simulink model "Charge_2_V1"  (R2017b)
settings: Solver=FixedStepDiscrete  StartTime=0.0  StopTime=1  FixedStep=0.001  RelTol=1e-3
PreLoadFcn:
  | librarySetup
  | eval([bdroot,'_startup']) %Calling [modelName]_startup.m
undefined symbols (not defined in the file or in its folder): A0, A1, Car1__Authorize, Car2_Authorize, CON2, CON3, CON4, Control_Mode_In, CurrentSP, D10, D12, D13, D2, D3, D4, D5, D6, D7, D8, Frequency_High_Point, Frequency_Low_Point, Frequency_Mid_high, Frequency_Mid_low, HVol_High_Point, HVol_Low_Point, HVol_Mid_high, HVol_Mid_low, HVoltage_Factor, SeconCar_ThreePhase, V_Current_five, V_Current_four, V_Current_one, V_Current_six, V_Current_three, V_Current_two, V_Frequency, V_MaxPliot, V_MinPliot, Vol_High_Point, Vol_Low_Point, Vol_Mid_high, Vol_Mid_low, Voltage_Factor, Voltage_Mode_Test
libraries: simulink x331, HANcoder_STM32_Target x30, powerlib_meascontrol x8, simulink_extras x2
(part 3 of 13)

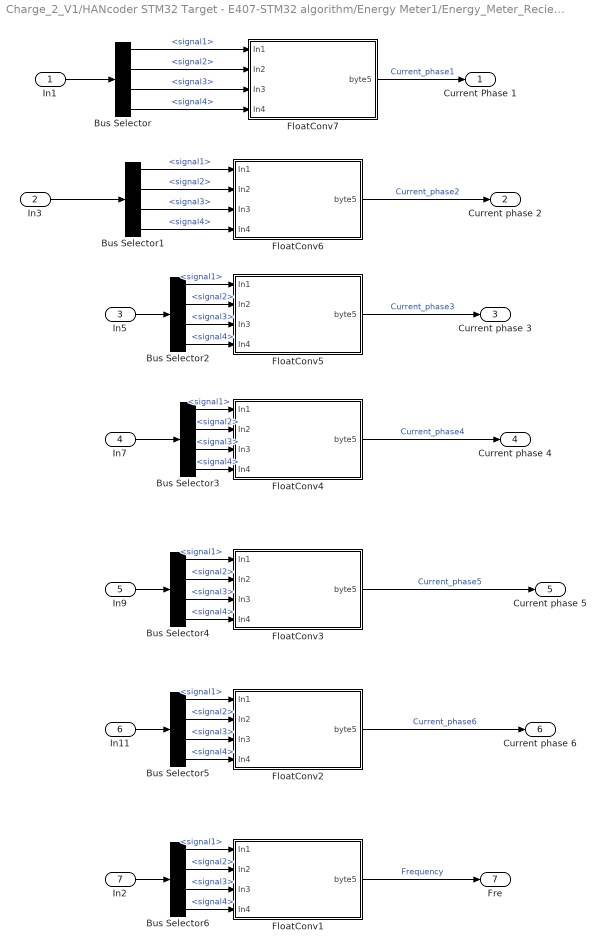
== system Charge_2_V1/HANcoder STM32 Target - E407-STM32 algorithm/Energy Meter1/Energy_Meter_Recieve/Subsystem ==
  In1 : Inport  SampleTime=0.1
  In3 : Inport  Port=2  SampleTime=0.1
  In5 : Inport  Port=3  SampleTime=0.1
  In7 : Inport  Port=4  SampleTime=0.1
  In9 : Inport  Port=5  SampleTime=0.1
  In11 : Inport  Port=6  SampleTime=0.1
  In2 : Inport  Port=7  SampleTime=0.1
  Bus Selector{,1..6} (7 alike) : BusSelector  OutputSignals=signal1,signal2,signal3,signal4
  FloatConv1 : Subsystem
  FloatConv2 : Subsystem
  FloatConv3 : Subsystem
  FloatConv4 : Subsystem
  FloatConv5 : Subsystem
  FloatConv6 : Subsystem
  FloatConv7 : Subsystem
  Current Phase 1 : Outport
  Current phase 2 : Outport  Port=2  SampleTime=0.1
  Current phase 3 : Outport  Port=3  SampleTime=0.1
  Current phase 4 : Outport  Port=4  SampleTime=0.1
  Current phase 5 : Outport  Port=5  SampleTime=0.1
  Current phase 6 : Outport  Port=6  SampleTime=0.1
  Fre : Outport  Port=7  SampleTime=0.1
  wires:
  FloatConv7/1(byte5) -> Current Phase 1/1  "Current_phase1"
  FloatConv6/1(byte5) -> Current phase 2/1  "Current_phase2"
  FloatConv5/1(byte5) -> Current phase 3/1  "Current_phase3"
  FloatConv4/1(byte5) -> Current phase 4/1  "Current_phase4"
  FloatConv3/1(byte5) -> Current phase 5/1  "Current_phase5"
  FloatConv2/1(byte5) -> Current phase 6/1  "Current_phase6"
  FloatConv1/1(byte5) -> Fre/1  "Frequency"
  In1/1 -> Bus Selector/1
  Bus Selector/1 -> FloatConv7/1(In1)  "<signal1>"
  Bus Selector/2 -> FloatConv7/2(In2)  "<signal2>"
  Bus Selector/3 -> FloatConv7/3(In3)  "<signal3>"
  Bus Selector/4 -> FloatConv7/4(In4)  "<signal4>"
  In3/1 -> Bus Selector1/1
  Bus Selector1/1 -> FloatConv6/1(In1)  "<signal1>"
  Bus Selector1/2 -> FloatConv6/2(In2)  "<signal2>"
  Bus Selector1/3 -> FloatConv6/3(In3)  "<signal3>"
  Bus Selector1/4 -> FloatConv6/4(In4)  "<signal4>"
  Bus Selector2/1 -> FloatConv5/1(In1)  "<signal1>"
  Bus Selector2/2 -> FloatConv5/2(In2)  "<signal2>"
  Bus Selector2/3 -> FloatConv5/3(In3)  "<signal3>"
  Bus Selector2/4 -> FloatConv5/4(In4)  "<signal4>"
  In5/1 -> Bus Selector2/1
  Bus Selector3/1 -> FloatConv4/1(In1)  "<signal1>"
  Bus Selector3/2 -> FloatConv4/2(In2)  "<signal2>"
  Bus Selector3/3 -> FloatConv4/3(In3)  "<signal3>"
  Bus Selector3/4 -> FloatConv4/4(In4)  "<signal4>"
  In7/1 -> Bus Selector3/1
  In9/1 -> Bus Selector4/1
  Bus Selector4/1 -> FloatConv3/1(In1)  "<signal1>"
  Bus Selector4/2 -> FloatConv3/2(In2)  "<signal2>"
  Bus Selector4/3 -> FloatConv3/3(In3)  "<signal3>"
  Bus Selector4/4 -> FloatConv3/4(In4)  "<signal4>"
  Bus Selector5/1 -> FloatConv2/1(In1)  "<signal1>"
  Bus Selector5/2 -> FloatConv2/2(In2)  "<signal2>"
  Bus Selector5/3 -> FloatConv2/3(In3)  "<signal3>"
  Bus Selector5/4 -> FloatConv2/4(In4)  "<signal4>"
  In11/1 -> Bus Selector5/1
  In2/1 -> Bus Selector6/1
  Bus Selector6/1 -> FloatConv1/1(In1)  "<signal1>"
  Bus Selector6/2 -> FloatConv1/2(In2)  "<signal2>"
  Bus Selector6/3 -> FloatConv1/3(In3)  "<signal3>"
  Bus Selector6/4 -> FloatConv1/4(In4)  "<signal4>"

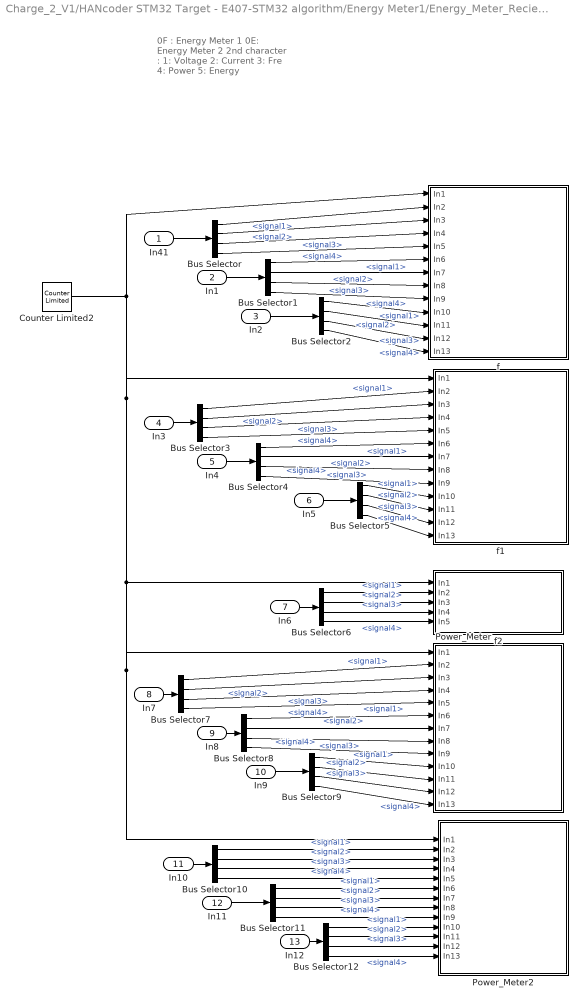
== system Charge_2_V1/HANcoder STM32 Target - E407-STM32 algorithm/Energy Meter1/Energy_Meter_Recieve/Subsystem1 ==
  note: 0F : Energy Meter 1
      | 0E: Energy Meter 2
      | 2nd character :
      | 1: Voltage
      | 2: Current
      | 3: Fre
      | 4: Power
      | 5: Energy
  In41 : Inport
  In1 : Inport  Port=2
  In2 : Inport  Port=3
  In3 : Inport  Port=4
  In4 : Inport  Port=5
  In5 : Inport  Port=6
  In6 : Inport  Port=7
  In7 : Inport  Port=8
  In8 : Inport  Port=9
  In9 : Inport  Port=10
  In10 : Inport  Port=11
  In11 : Inport  Port=12
  In12 : Inport  Port=13
  Bus Selector{,1..12} (13 alike) : BusSelector  OutputSignals=signal1,signal2,signal3,signal4
  Counter Limited2 : simulink/Sources/Counter Limited  uplimit=1200  tsamp=0.001
  Power_Meter : Subsystem
  Power_Meter2 : Subsystem
  f : Subsystem
  f1 : Subsystem
  f2 : Subsystem
  wires:
  Counter Limited2/1 -> f/1(In1), Power_Meter2/1(In1), Power_Meter/1(In1), f2/1(In1), f1/1(In1)
  In41/1 -> Bus Selector/1
  Bus Selector/1 -> f/2(In2)  "<signal1>"
  Bus Selector/2 -> f/3(In3)  "<signal2>"
  Bus Selector/3 -> f/4(In4)  "<signal3>"
  Bus Selector/4 -> f/5(In5)  "<signal4>"
  In1/1 -> Bus Selector1/1
  Bus Selector1/1 -> f/6(In6)  "<signal1>"
  Bus Selector1/2 -> f/7(In7)  "<signal2>"
  Bus Selector1/3 -> f/8(In8)  "<signal3>"
  Bus Selector1/4 -> f/9(In9)  "<signal4>"
  Bus Selector2/1 -> f/10(In10)  "<signal1>"
  Bus Selector2/2 -> f/11(In11)  "<signal2>"
  Bus Selector2/3 -> f/12(In12)  "<signal3>"
  Bus Selector2/4 -> f/13(In13)  "<signal4>"
  In2/1 -> Bus Selector2/1
  Bus Selector3/1 -> f1/2(In2)  "<signal1>"
  Bus Selector3/2 -> f1/3(In3)  "<signal2>"
  Bus Selector3/3 -> f1/4(In4)  "<signal3>"
  Bus Selector3/4 -> f1/5(In5)  "<signal4>"
  In3/1 -> Bus Selector3/1
  Bus Selector4/1 -> f1/6(In6)  "<signal1>"
  Bus Selector4/2 -> f1/7(In7)  "<signal2>"
  Bus Selector4/3 -> f1/8(In8)  "<signal3>"
  Bus Selector4/4 -> f1/9(In9)  "<signal4>"
  In4/1 -> Bus Selector4/1
  Bus Selector5/2 -> f1/11(In11)  "<signal2>"
  Bus Selector5/3 -> f1/12(In12)  "<signal3>"
  Bus Selector5/4 -> f1/13(In13)  "<signal4>"
  Bus Selector5/1 -> f1/10(In10)  "<signal1>"
  In5/1 -> Bus Selector5/1
  In6/1 -> Bus Selector6/1
  Bus Selector7/1 -> Power_Meter/2(In2)  "<signal1>"
  Bus Selector7/2 -> Power_Meter/3(In3)  "<signal2>"
  Bus Selector7/3 -> Power_Meter/4(In4)  "<signal3>"
  Bus Selector7/4 -> Power_Meter/5(In5)  "<signal4>"
  Bus Selector8/1 -> Power_Meter/6(In6)  "<signal1>"
  Bus Selector8/2 -> Power_Meter/7(In7)  "<signal2>"
  Bus Selector8/3 -> Power_Meter/8(In8)  "<signal3>"
  Bus Selector8/4 -> Power_Meter/9(In9)  "<signal4>"
  Bus Selector9/1 -> Power_Meter/10(In10)  "<signal1>"
  Bus Selector9/2 -> Power_Meter/11(In11)  "<signal2>"
  Bus Selector9/3 -> Power_Meter/12(In12)  "<signal3>"
  Bus Selector9/4 -> Power_Meter/13(In13)  "<signal4>"
  In7/1 -> Bus Selector7/1
  In8/1 -> Bus Selector8/1
  In9/1 -> Bus Selector9/1
  Bus Selector11/1 -> Power_Meter2/6(In6)  "<signal1>"
  Bus Selector11/2 -> Power_Meter2/7(In7)  "<signal2>"
  Bus Selector11/3 -> Power_Meter2/8(In8)  "<signal3>"
  Bus Selector11/4 -> Power_Meter2/9(In9)  "<signal4>"
  Bus Selector12/1 -> Power_Meter2/10(In10)  "<signal1>"
  Bus Selector12/2 -> Power_Meter2/11(In11)  "<signal2>"
  Bus Selector12/3 -> Power_Meter2/12(In12)  "<signal3>"
  Bus Selector12/4 -> Power_Meter2/13(In13)  "<signal4>"
  In10/1 -> Bus Selector10/1
  In11/1 -> Bus Selector11/1
  In12/1 -> Bus Selector12/1
  Bus Selector6/1 -> f2/2(In2)  "<signal1>"
  Bus Selector6/2 -> f2/3(In3)  "<signal2>"
  Bus Selector6/3 -> f2/4(In4)  "<signal3>"
  Bus Selector6/4 -> f2/5(In5)  "<signal4>"
  Bus Selector10/1 -> Power_Meter2/2(In2)  "<signal1>"
  Bus Selector10/2 -> Power_Meter2/3(In3)  "<signal2>"
  Bus Selector10/3 -> Power_Meter2/4(In4)  "<signal3>"
  Bus Selector10/4 -> Power_Meter2/5(In5)  "<signal4>"

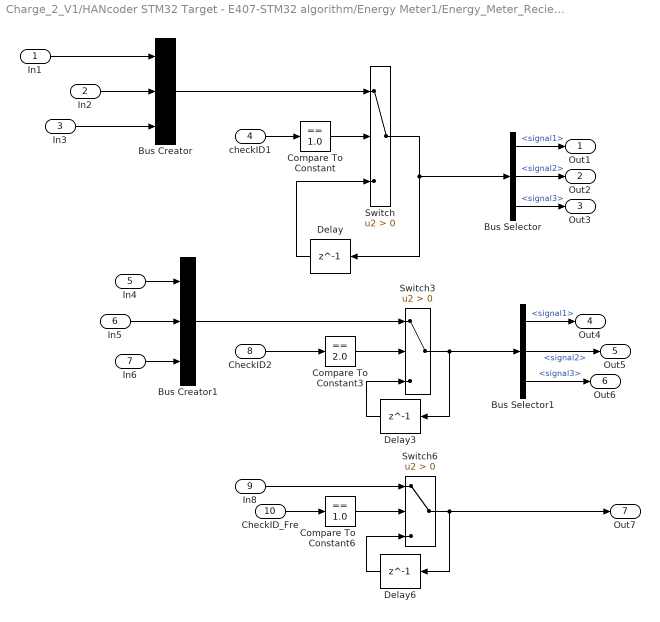
== system Charge_2_V1/HANcoder STM32 Target - E407-STM32 algorithm/Energy Meter1/Energy_Meter_Recieve/Subsystem2 ==
  In1 : Inport
  In2 : Inport  Port=2
  In3 : Inport  Port=3
  checkID1 : Inport  Port=4
  In4 : Inport  Port=5
  In5 : Inport  Port=6
  In6 : Inport  Port=7
  CheckID2 : Inport  Port=8
  In8 : Inport  Port=9
  CheckID_Fre : Inport  Port=10
  Bus Creator : BusCreator  Inputs=3
  Bus Creator1 : BusCreator  Inputs=3
  Bus Selector : BusSelector  OutputSignals=signal1,signal2,signal3
  Bus Selector1 : BusSelector  OutputSignals=signal1,signal2,signal3
  Compare To Constant : simulink/Logic and Bit Operations/Compare To Constant  relop===  const=1.0  OutDataTypeStr=boolean
  Compare To Constant3 : simulink/Logic and Bit Operations/Compare To Constant  relop===  const=2.0  OutDataTypeStr=boolean
  Compare To Constant6 : simulink/Logic and Bit Operations/Compare To Constant  relop===  const=1.0  OutDataTypeStr=boolean
  Delay : Delay  DelayLength=1  InitialCondition=0
  Delay3 : Delay  DelayLength=1  InitialCondition=0
  Delay6 : Delay  DelayLength=1  InitialCondition=0
  Switch : Switch  Criteria=u2 > Threshold
  Switch3 : Switch  Criteria=u2 > Threshold
  Switch6 : Switch  Criteria=u2 > Threshold
  Out1 : Outport
  Out2 : Outport  Port=2
  Out3 : Outport  Port=3
  Out4 : Outport  Port=4
  Out5 : Outport  Port=5
  Out6 : Outport  Port=6
  Out7 : Outport  Port=7
  wires:
  Compare To Constant/1 -> Switch/2
  Switch/1 -> Delay/1, Bus Selector/1
  In1/1 -> Bus Creator/1
  Delay/1 -> Switch/3
  Switch3/1 -> Delay3/1, Bus Selector1/1
  Compare To Constant3/1 -> Switch3/2
  Delay3/1 -> Switch3/3
  Switch6/1 -> Out7/1, Delay6/1
  Compare To Constant6/1 -> Switch6/2
  Delay6/1 -> Switch6/3
  In2/1 -> Bus Creator/2
  In3/1 -> Bus Creator/3
  Bus Creator/1 -> Switch/1
  Bus Creator1/1 -> Switch3/1
  checkID1/1 -> Compare To Constant/1
  In8/1 -> Switch6/1
  Bus Selector/1 -> Out1/1  "<signal1>"
  Bus Selector/2 -> Out2/1  "<signal2>"
  Bus Selector/3 -> Out3/1  "<signal3>"
  In4/1 -> Bus Creator1/1
  In5/1 -> Bus Creator1/2
  In6/1 -> Bus Creator1/3
  CheckID2/1 -> Compare To Constant3/1
  CheckID_Fre/1 -> Compare To Constant6/1
  Bus Selector1/1 -> Out4/1  "<signal1>"
  Bus Selector1/2 -> Out5/1  "<signal2>"
  Bus Selector1/3 -> Out6/1  "<signal3>"

== system Charge_2_V1/HANcoder STM32 Target - E407-STM32 algorithm/Energy Meter1/Energy_Meter_Recieve/Subsystem3 ==
  In1 : Inport
  In2 : Inport  Port=2
  In3 : Inport  Port=3
  checkID1 : Inport  Port=4
  In4 : Inport  Port=5
  In5 : Inport  Port=6
  In6 : Inport  Port=7
  CheckID2 : Inport  Port=8
  Bus Creator : BusCreator  Inputs=3
  Bus Creator1 : BusCreator  Inputs=3
  Bus Selector : BusSelector  OutputSignals=signal1,signal2,signal3
  Bus Selector1 : BusSelector  OutputSignals=signal1,signal2,signal3
  Compare To Constant : simulink/Logic and Bit Operations/Compare To Constant  relop===  const=1.0  OutDataTypeStr=boolean
  Compare To Constant3 : simulink/Logic and Bit Operations/Compare To Constant  relop===  const=2.0  OutDataTypeStr=boolean
  Delay : Delay  DelayLength=1  InitialCondition=0
  Delay3 : Delay  DelayLength=1  InitialCondition=0
  Switch : Switch  Criteria=u2 > Threshold
  Switch3 : Switch  Criteria=u2 > Threshold
  Out1 : Outport
  Out2 : Outport  Port=2
  Out3 : Outport  Port=3
  Out4 : Outport  Port=4
  Out5 : Outport  Port=5
  Out6 : Outport  Port=6
  wires:
  Compare To Constant/1 -> Switch/2
  Switch/1 -> Delay/1, Bus Selector/1
  In1/1 -> Bus Creator/1
  Delay/1 -> Switch/3
  Switch3/1 -> Delay3/1, Bus Selector1/1
  Compare To Constant3/1 -> Switch3/2
  Delay3/1 -> Switch3/3
  In2/1 -> Bus Creator/2
  In3/1 -> Bus Creator/3
  Bus Creator/1 -> Switch/1
  Bus Creator1/1 -> Switch3/1
  checkID1/1 -> Compare To Constant/1
  Bus Selector/1 -> Out1/1  "<signal1>"
  Bus Selector/2 -> Out2/1  "<signal2>"
  Bus Selector/3 -> Out3/1  "<signal3>"
  In4/1 -> Bus Creator1/1
  In5/1 -> Bus Creator1/2
  In6/1 -> Bus Creator1/3
  CheckID2/1 -> Compare To Constant3/1
  Bus Selector1/1 -> Out4/1  "<signal1>"
  Bus Selector1/2 -> Out5/1  "<signal2>"
  Bus Selector1/3 -> Out6/1  "<signal3>"

== system Charge_2_V1/HANcoder STM32 Target - E407-STM32 algorithm/Energy Meter1/Energy_Meter_Recieve/Subsystem5 ==
  In1 : Inport  SampleTime=0.1
  In3 : Inport  Port=2  SampleTime=0.1
  In5 : Inport  Port=3  SampleTime=0.1
  In7 : Inport  Port=4  SampleTime=0.1
  In9 : Inport  Port=5  SampleTime=0.1
  In11 : Inport  Port=6  SampleTime=0.1
  Bus Selector{,1..5} (6 alike) : BusSelector  OutputSignals=signal1,signal2,signal3,signal4
  FloatConv2 : Subsystem
  FloatConv3 : Subsystem
  FloatConv4 : Subsystem
  FloatConv5 : Subsystem
  FloatConv6 : Subsystem
  FloatConv7 : Subsystem
  Voltage1 : Outport
  Voltage2 : Outport  Port=2  SampleTime=0.1
  Voltage3 : Outport  Port=3  SampleTime=0.1
  Voltage4 : Outport  Port=4  SampleTime=0.1
  Voltage5 : Outport  Port=5  SampleTime=0.1
  Voltage6 : Outport  Port=6  SampleTime=0.1
  wires:
  In11/1 -> Bus Selector5/1
  Bus Selector5/4 -> FloatConv2/4(In4)  "<signal4>"
  Bus Selector5/3 -> FloatConv2/3(In3)  "<signal3>"
  Bus Selector5/2 -> FloatConv2/2(In2)  "<signal2>"
  Bus Selector5/1 -> FloatConv2/1(In1)  "<signal1>"
  Bus Selector4/4 -> FloatConv3/4(In4)  "<signal4>"
  Bus Selector4/3 -> FloatConv3/3(In3)  "<signal3>"
  Bus Selector4/2 -> FloatConv3/2(In2)  "<signal2>"
  Bus Selector4/1 -> FloatConv3/1(In1)  "<signal1>"
  In9/1 -> Bus Selector4/1
  In7/1 -> Bus Selector3/1
  Bus Selector3/4 -> FloatConv4/4(In4)  "<signal4>"
  Bus Selector3/3 -> FloatConv4/3(In3)  "<signal3>"
  Bus Selector3/2 -> FloatConv4/2(In2)  "<signal2>"
  Bus Selector3/1 -> FloatConv4/1(In1)  "<signal1>"
  In5/1 -> Bus Selector2/1
  Bus Selector2/4 -> FloatConv5/4(In4)  "<signal4>"
  Bus Selector2/3 -> FloatConv5/3(In3)  "<signal3>"
  Bus Selector2/2 -> FloatConv5/2(In2)  "<signal2>"
  Bus Selector2/1 -> FloatConv5/1(In1)  "<signal1>"
  Bus Selector1/4 -> FloatConv6/4(In4)  "<signal4>"
  Bus Selector1/3 -> FloatConv6/3(In3)  "<signal3>"
  Bus Selector1/2 -> FloatConv6/2(In2)  "<signal2>"
  Bus Selector1/1 -> FloatConv6/1(In1)  "<signal1>"
  In3/1 -> Bus Selector1/1
  Bus Selector/4 -> FloatConv7/4(In4)  "<signal4>"
  Bus Selector/3 -> FloatConv7/3(In3)  "<signal3>"
  Bus Selector/2 -> FloatConv7/2(In2)  "<signal2>"
  Bus Selector/1 -> FloatConv7/1(In1)  "<signal1>"
  In1/1 -> Bus Selector/1
  FloatConv2/1(byte5) -> Voltage6/1  "Voltage_phase6"
  FloatConv3/1(byte5) -> Voltage5/1  "Voltage_phase5"
  FloatConv4/1(byte5) -> Voltage4/1  "Voltage_phase4"
  FloatConv5/1(byte5) -> Voltage3/1  "Voltage_phase3"
  FloatConv6/1(byte5) -> Voltage2/1  "Voltage_phase2"
  FloatConv7/1(byte5) -> Voltage1/1  "Voltage_phase1"

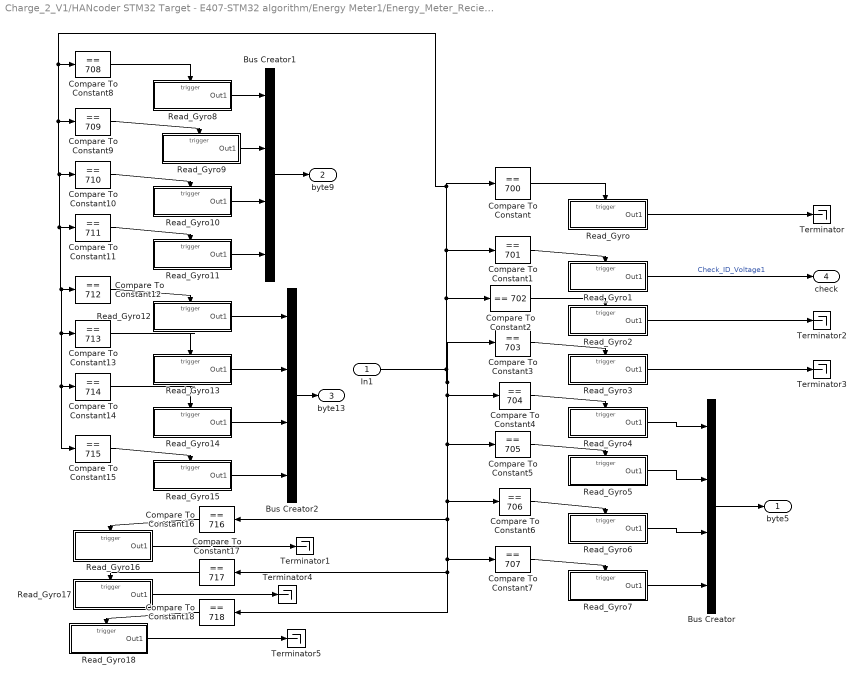
== system Charge_2_V1/HANcoder STM32 Target - E407-STM32 algorithm/Energy Meter1/Energy_Meter_Recieve/Voltage_Meter_1 ==
  In1 : Inport
  Bus Creator : BusCreator  Inputs=4
  Bus Creator1 : BusCreator  Inputs=4
  Bus Creator2 : BusCreator  Inputs=4
  Compare To Constant : simulink/Logic and Bit Operations/Compare To Constant  relop===  const=700  OutDataTypeStr=uint8
  Compare To Constant1 : simulink/Logic and Bit Operations/Compare To Constant  relop===  const=701  OutDataTypeStr=uint8
  Compare To Constant10 : simulink/Logic and Bit Operations/Compare To Constant  relop===  const=710  OutDataTypeStr=uint8
  Compare To Constant11 : simulink/Logic and Bit Operations/Compare To Constant  relop===  const=711  OutDataTypeStr=uint8
  Compare To Constant12 : simulink/Logic and Bit Operations/Compare To Constant  relop===  const=712  OutDataTypeStr=uint8
  Compare To Constant13 : simulink/Logic and Bit Operations/Compare To Constant  relop===  const=713  OutDataTypeStr=uint8
  Compare To Constant14 : simulink/Logic and Bit Operations/Compare To Constant  relop===  const=714  OutDataTypeStr=uint8
  Compare To Constant15 : simulink/Logic and Bit Operations/Compare To Constant  relop===  const=715  OutDataTypeStr=uint8
  Compare To Constant16 : simulink/Logic and Bit Operations/Compare To Constant  relop===  const=716  OutDataTypeStr=uint8
  Compare To Constant17 : simulink/Logic and Bit Operations/Compare To Constant  relop===  const=717  OutDataTypeStr=uint8
  Compare To Constant18 : simulink/Logic and Bit Operations/Compare To Constant  relop===  const=718  OutDataTypeStr=uint8
  Compare To Constant2 : simulink/Logic and Bit Operations/Compare To Constant  relop===  const=702  OutDataTypeStr=uint8
  Compare To Constant3 : simulink/Logic and Bit Operations/Compare To Constant  relop===  const=703  OutDataTypeStr=uint8
  Compare To Constant4 : simulink/Logic and Bit Operations/Compare To Constant  relop===  const=704  OutDataTypeStr=uint8
  Compare To Constant5 : simulink/Logic and Bit Operations/Compare To Constant  relop===  const=705  OutDataTypeStr=uint8
  Compare To Constant6 : simulink/Logic and Bit Operations/Compare To Constant  relop===  const=706  OutDataTypeStr=uint8
  Compare To Constant7 : simulink/Logic and Bit Operations/Compare To Constant  relop===  const=707  OutDataTypeStr=uint8
  Compare To Constant8 : simulink/Logic and Bit Operations/Compare To Constant  relop===  const=708  OutDataTypeStr=uint8
  Compare To Constant9 : simulink/Logic and Bit Operations/Compare To Constant  relop===  const=709  OutDataTypeStr=uint8
  Read_Gyro : Subsystem  TreatAsAtomicUnit=on
  Read_Gyro1 : Subsystem  TreatAsAtomicUnit=on
  Read_Gyro10 : Subsystem  TreatAsAtomicUnit=on
  Read_Gyro11 : Subsystem  TreatAsAtomicUnit=on
  Read_Gyro12 : Subsystem  TreatAsAtomicUnit=on
  Read_Gyro13 : Subsystem  TreatAsAtomicUnit=on
  Read_Gyro14 : Subsystem  TreatAsAtomicUnit=on
  Read_Gyro15 : Subsystem  TreatAsAtomicUnit=on
  Read_Gyro16 : Subsystem  TreatAsAtomicUnit=on
  Read_Gyro17 : Subsystem  TreatAsAtomicUnit=on
  Read_Gyro18 : Subsystem  TreatAsAtomicUnit=on
  Read_Gyro2 : Subsystem  TreatAsAtomicUnit=on
  Read_Gyro3 : Subsystem  TreatAsAtomicUnit=on
  Read_Gyro4 : Subsystem  TreatAsAtomicUnit=on
  Read_Gyro5 : Subsystem  TreatAsAtomicUnit=on
  Read_Gyro6 : Subsystem  TreatAsAtomicUnit=on
  Read_Gyro7 : Subsystem  TreatAsAtomicUnit=on
  Read_Gyro8 : Subsystem  TreatAsAtomicUnit=on
  Read_Gyro9 : Subsystem  TreatAsAtomicUnit=on
  Terminator{,1..5} (6 alike) : Terminator
  byte5 : Outport
  byte9 : Outport  Port=2
  byte13 : Outport  Port=3
  check : Outport  Port=4
  wires:
  Bus Creator2/1 -> byte13/1
  Read_Gyro15/1(Out1) -> Bus Creator2/4
  Read_Gyro14/1(Out1) -> Bus Creator2/3
  Read_Gyro12/1(Out1) -> Bus Creator2/1
  Read_Gyro13/1(Out1) -> Bus Creator2/2
  Bus Creator1/1 -> byte9/1
  Read_Gyro11/1(Out1) -> Bus Creator1/4
  Read_Gyro10/1(Out1) -> Bus Creator1/3
  Read_Gyro9/1(Out1) -> Bus Creator1/2
  Read_Gyro8/1(Out1) -> Bus Creator1/1
  Bus Creator/1 -> byte5/1
  Read_Gyro6/1(Out1) -> Bus Creator/3
  Read_Gyro5/1(Out1) -> Bus Creator/2
  Read_Gyro7/1(Out1) -> Bus Creator/4
  Read_Gyro4/1(Out1) -> Bus Creator/1
  Read_Gyro1/1(Out1) -> check/1  "Check_ID_Voltage1"
  Compare To Constant2/1 -> Read_Gyro2/Trigger
  Compare To Constant1/1 -> Read_Gyro1/Trigger
  Read_Gyro/1(Out1) -> Terminator/1
  Compare To Constant/1 -> Read_Gyro/Trigger
  Compare To Constant4/1 -> Read_Gyro4/Trigger
  Compare To Constant6/1 -> Read_Gyro6/Trigger
  Compare To Constant9/1 -> Read_Gyro9/Trigger
  Read_Gyro3/1(Out1) -> Terminator3/1
  Read_Gyro2/1(Out1) -> Terminator2/1
  Compare To Constant3/1 -> Read_Gyro3/Trigger
  Compare To Constant7/1 -> Read_Gyro7/Trigger
  Compare To Constant5/1 -> Read_Gyro5/Trigger
  Compare To Constant10/1 -> Read_Gyro10/Trigger
  Compare To Constant11/1 -> Read_Gyro11/Trigger
  Compare To Constant12/1 -> Read_Gyro12/Trigger
  Compare To Constant13/1 -> Read_Gyro13/Trigger
  In1/1 -> Compare To Constant17/1, Compare To Constant18/1, Compare To Constant7/1, Compare To Constant16/1, Compare To Constant6/1, Compare To Constant5/1, Compare To Constant4/1, Compare To Constant3/1, Compare To Constant/1, Compare To Constant8/1, Compare To Constant9/1, Compare To Constant10/1, Compare To Constant11/1, Compare To Constant12/1, Compare To Constant13/1, Compare To Constant14/1, Compare To Constant15/1, Compare To Constant1/1, Compare To Constant2/1
  Compare To Constant8/1 -> Read_Gyro8/Trigger
  Compare To Constant14/1 -> Read_Gyro14/Trigger
  Compare To Constant15/1 -> Read_Gyro15/Trigger
  Compare To Constant16/1 -> Read_Gyro16/Trigger
  Compare To Constant17/1 -> Read_Gyro17/Trigger
  Compare To Constant18/1 -> Read_Gyro18/Trigger
  Read_Gyro16/1(Out1) -> Terminator1/1
  Read_Gyro17/1(Out1) -> Terminator4/1
  Read_Gyro18/1(Out1) -> Terminator5/1

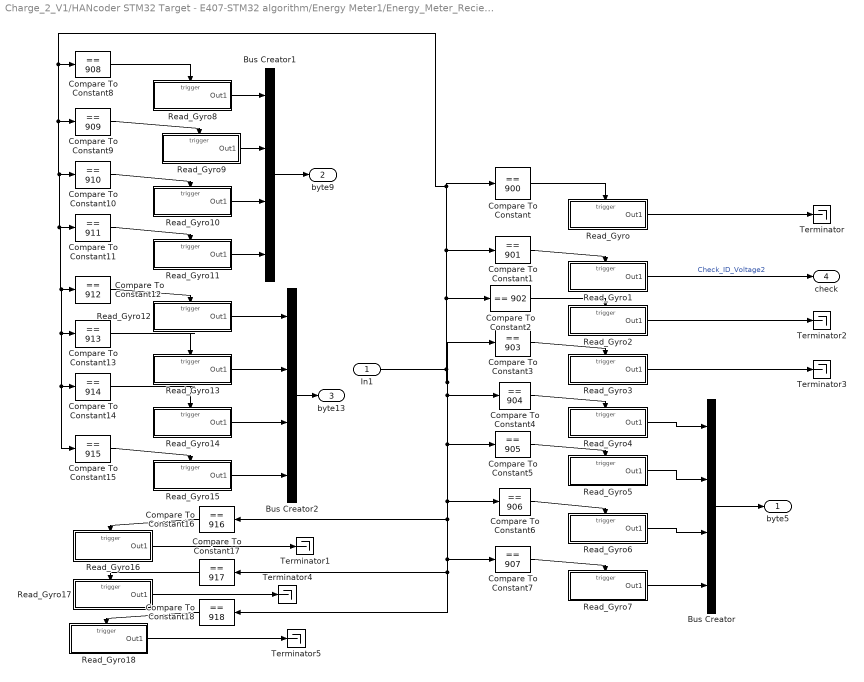
== system Charge_2_V1/HANcoder STM32 Target - E407-STM32 algorithm/Energy Meter1/Energy_Meter_Recieve/Voltage_Meter_2 ==
  In1 : Inport
  Bus Creator : BusCreator  Inputs=4
  Bus Creator1 : BusCreator  Inputs=4
  Bus Creator2 : BusCreator  Inputs=4
  Compare To Constant : simulink/Logic and Bit Operations/Compare To Constant  relop===  const=900  OutDataTypeStr=uint8
  Compare To Constant1 : simulink/Logic and Bit Operations/Compare To Constant  relop===  const=901  OutDataTypeStr=uint8
  Compare To Constant10 : simulink/Logic and Bit Operations/Compare To Constant  relop===  const=910  OutDataTypeStr=uint8
  Compare To Constant11 : simulink/Logic and Bit Operations/Compare To Constant  relop===  const=911  OutDataTypeStr=uint8
  Compare To Constant12 : simulink/Logic and Bit Operations/Compare To Constant  relop===  const=912  OutDataTypeStr=uint8
  Compare To Constant13 : simulink/Logic and Bit Operations/Compare To Constant  relop===  const=913  OutDataTypeStr=uint8
  Compare To Constant14 : simulink/Logic and Bit Operations/Compare To Constant  relop===  const=914  OutDataTypeStr=uint8
  Compare To Constant15 : simulink/Logic and Bit Operations/Compare To Constant  relop===  const=915  OutDataTypeStr=uint8
  Compare To Constant16 : simulink/Logic and Bit Operations/Compare To Constant  relop===  const=916  OutDataTypeStr=uint8
  Compare To Constant17 : simulink/Logic and Bit Operations/Compare To Constant  relop===  const=917  OutDataTypeStr=uint8
  Compare To Constant18 : simulink/Logic and Bit Operations/Compare To Constant  relop===  const=918  OutDataTypeStr=uint8
  Compare To Constant2 : simulink/Logic and Bit Operations/Compare To Constant  relop===  const=902  OutDataTypeStr=uint8
  Compare To Constant3 : simulink/Logic and Bit Operations/Compare To Constant  relop===  const=903  OutDataTypeStr=uint8
  Compare To Constant4 : simulink/Logic and Bit Operations/Compare To Constant  relop===  const=904  OutDataTypeStr=uint8
  Compare To Constant5 : simulink/Logic and Bit Operations/Compare To Constant  relop===  const=905  OutDataTypeStr=uint8
  Compare To Constant6 : simulink/Logic and Bit Operations/Compare To Constant  relop===  const=906  OutDataTypeStr=uint8
  Compare To Constant7 : simulink/Logic and Bit Operations/Compare To Constant  relop===  const=907  OutDataTypeStr=uint8
  Compare To Constant8 : simulink/Logic and Bit Operations/Compare To Constant  relop===  const=908  OutDataTypeStr=uint8
  Compare To Constant9 : simulink/Logic and Bit Operations/Compare To Constant  relop===  const=909  OutDataTypeStr=uint8
  Read_Gyro : Subsystem  TreatAsAtomicUnit=on
  Read_Gyro1 : Subsystem  TreatAsAtomicUnit=on
  Read_Gyro10 : Subsystem  TreatAsAtomicUnit=on
  Read_Gyro11 : Subsystem  TreatAsAtomicUnit=on
  Read_Gyro12 : Subsystem  TreatAsAtomicUnit=on
  Read_Gyro13 : Subsystem  TreatAsAtomicUnit=on
  Read_Gyro14 : Subsystem  TreatAsAtomicUnit=on
  Read_Gyro15 : Subsystem  TreatAsAtomicUnit=on
  Read_Gyro16 : Subsystem  TreatAsAtomicUnit=on
  Read_Gyro17 : Subsystem  TreatAsAtomicUnit=on
  Read_Gyro18 : Subsystem  TreatAsAtomicUnit=on
  Read_Gyro2 : Subsystem  TreatAsAtomicUnit=on
  Read_Gyro3 : Subsystem  TreatAsAtomicUnit=on
  Read_Gyro4 : Subsystem  TreatAsAtomicUnit=on
  Read_Gyro5 : Subsystem  TreatAsAtomicUnit=on
  Read_Gyro6 : Subsystem  TreatAsAtomicUnit=on
  Read_Gyro7 : Subsystem  TreatAsAtomicUnit=on
  Read_Gyro8 : Subsystem  TreatAsAtomicUnit=on
  Read_Gyro9 : Subsystem  TreatAsAtomicUnit=on
  Terminator{,1..5} (6 alike) : Terminator
  byte5 : Outport
  byte9 : Outport  Port=2
  byte13 : Outport  Port=3
  check : Outport  Port=4
  wires:
  Read_Gyro18/1(Out1) -> Terminator5/1
  Read_Gyro17/1(Out1) -> Terminator4/1
  Read_Gyro16/1(Out1) -> Terminator1/1
  Compare To Constant18/1 -> Read_Gyro18/Trigger
  Compare To Constant17/1 -> Read_Gyro17/Trigger
  Compare To Constant16/1 -> Read_Gyro16/Trigger
  Compare To Constant15/1 -> Read_Gyro15/Trigger
  Compare To Constant14/1 -> Read_Gyro14/Trigger
  Compare To Constant8/1 -> Read_Gyro8/Trigger
  In1/1 -> Compare To Constant2/1, Compare To Constant1/1, Compare To Constant15/1, Compare To Constant14/1, Compare To Constant13/1, Compare To Constant12/1, Compare To Constant11/1, Compare To Constant10/1, Compare To Constant9/1, Compare To Constant8/1, Compare To Constant/1, Compare To Constant3/1, Compare To Constant4/1, Compare To Constant5/1, Compare To Constant6/1, Compare To Constant16/1, Compare To Constant7/1, Compare To Constant18/1, Compare To Constant17/1
  Compare To Constant13/1 -> Read_Gyro13/Trigger
  Compare To Constant12/1 -> Read_Gyro12/Trigger
  Compare To Constant11/1 -> Read_Gyro11/Trigger
  Compare To Constant10/1 -> Read_Gyro10/Trigger
  Compare To Constant5/1 -> Read_Gyro5/Trigger
  Compare To Constant7/1 -> Read_Gyro7/Trigger
  Compare To Constant3/1 -> Read_Gyro3/Trigger
  Read_Gyro2/1(Out1) -> Terminator2/1
  Read_Gyro3/1(Out1) -> Terminator3/1
  Compare To Constant9/1 -> Read_Gyro9/Trigger
  Compare To Constant6/1 -> Read_Gyro6/Trigger
  Compare To Constant4/1 -> Read_Gyro4/Trigger
  Compare To Constant/1 -> Read_Gyro/Trigger
  Read_Gyro/1(Out1) -> Terminator/1
  Compare To Constant1/1 -> Read_Gyro1/Trigger
  Compare To Constant2/1 -> Read_Gyro2/Trigger
  Read_Gyro1/1(Out1) -> check/1  "Check_ID_Voltage2"
  Read_Gyro4/1(Out1) -> Bus Creator/1
  Read_Gyro7/1(Out1) -> Bus Creator/4
  Read_Gyro5/1(Out1) -> Bus Creator/2
  Read_Gyro6/1(Out1) -> Bus Creator/3
  Bus Creator/1 -> byte5/1
  Read_Gyro8/1(Out1) -> Bus Creator1/1
  Read_Gyro9/1(Out1) -> Bus Creator1/2
  Read_Gyro10/1(Out1) -> Bus Creator1/3
  Read_Gyro11/1(Out1) -> Bus Creator1/4
  Bus Creator1/1 -> byte9/1
  Read_Gyro13/1(Out1) -> Bus Creator2/2
  Read_Gyro12/1(Out1) -> Bus Creator2/1
  Read_Gyro14/1(Out1) -> Bus Creator2/3
  Read_Gyro15/1(Out1) -> Bus Creator2/4
  Bus Creator2/1 -> byte13/1

== system Charge_2_V1/HANcoder STM32 Target - E407-STM32 algorithm/Energy Meter1/Energymeter_Request/Current_Meter_1  ==
  In1 : Inport
  Compare To Constant : simulink/Logic and Bit Operations/Compare To Constant  relop===  const=1  OutDataTypeStr=boolean
  Compare To Constant1 : simulink/Logic and Bit Operations/Compare To Constant  relop===  const=2  OutDataTypeStr=boolean
  Compare To Constant2 : simulink/Logic and Bit Operations/Compare To Constant  relop===  const=3  OutDataTypeStr=boolean
  Compare To Constant3 : simulink/Logic and Bit Operations/Compare To Constant  relop===  const=4  OutDataTypeStr=boolean
  Compare To Constant4 : simulink/Logic and Bit Operations/Compare To Constant  relop===  const=5  OutDataTypeStr=boolean
  Compare To Constant5 : simulink/Logic and Bit Operations/Compare To Constant  relop===  const=6  OutDataTypeStr=boolean
  Compare To Constant6 : simulink/Logic and Bit Operations/Compare To Constant  relop===  const=7  OutDataTypeStr=boolean
  Compare To Constant7 : simulink/Logic and Bit Operations/Compare To Constant  relop===  const=8  OutDataTypeStr=boolean
  Read_Gyro1 : Subsystem  TreatAsAtomicUnit=on
  Read_Gyro2 : Subsystem  TreatAsAtomicUnit=on
  Read_Gyro3 : Subsystem  TreatAsAtomicUnit=on
  Read_Gyro4 : Subsystem  TreatAsAtomicUnit=on
  Read_Gyro5 : Subsystem  TreatAsAtomicUnit=on
  Read_Gyro6 : Subsystem  TreatAsAtomicUnit=on
  Read_Gyro7 : Subsystem  TreatAsAtomicUnit=on
  Read_Gyro8 : Subsystem  TreatAsAtomicUnit=on
  wires:
  In1/1 -> Compare To Constant7/1, Compare To Constant6/1, Compare To Constant5/1, Compare To Constant4/1, Compare To Constant3/1, Compare To Constant2/1, Compare To Constant1/1, Compare To Constant/1
  Compare To Constant7/1 -> Read_Gyro8/Trigger
  Compare To Constant6/1 -> Read_Gyro7/Trigger
  Compare To Constant5/1 -> Read_Gyro6/Trigger
  Compare To Constant4/1 -> Read_Gyro5/Trigger
  Compare To Constant/1 -> Read_Gyro1/Trigger  "counter"
  Compare To Constant2/1 -> Read_Gyro3/Trigger
  Compare To Constant1/1 -> Read_Gyro2/Trigger
  Compare To Constant3/1 -> Read_Gyro4/Trigger

== system Charge_2_V1/HANcoder STM32 Target - E407-STM32 algorithm/Energy Meter1/Energymeter_Request/Current_Meter_2 ==
  In1 : Inport
  Compare To Constant10 : simulink/Logic and Bit Operations/Compare To Constant  relop===  const=202  OutDataTypeStr=boolean
  Compare To Constant12 : simulink/Logic and Bit Operations/Compare To Constant  relop===  const=203  OutDataTypeStr=boolean
  Compare To Constant13 : simulink/Logic and Bit Operations/Compare To Constant  relop===  const=204  OutDataTypeStr=boolean
  Compare To Constant14 : simulink/Logic and Bit Operations/Compare To Constant  relop===  const=205  OutDataTypeStr=boolean
  Compare To Constant15 : simulink/Logic and Bit Operations/Compare To Constant  relop===  const=206  OutDataTypeStr=boolean
  Compare To Constant16 : simulink/Logic and Bit Operations/Compare To Constant  relop===  const=207  OutDataTypeStr=boolean
  Compare To Constant17 : simulink/Logic and Bit Operations/Compare To Constant  relop===  const=208  OutDataTypeStr=boolean
  Compare To Constant8 : simulink/Logic and Bit Operations/Compare To Constant  relop===  const=201  OutDataTypeStr=boolean
  Read_Gyro10 : Subsystem  TreatAsAtomicUnit=on
  Read_Gyro11 : Subsystem  TreatAsAtomicUnit=on
  Read_Gyro12 : Subsystem  TreatAsAtomicUnit=on
  Read_Gyro13 : Subsystem  TreatAsAtomicUnit=on
  Read_Gyro14 : Subsystem  TreatAsAtomicUnit=on
  Read_Gyro15 : Subsystem  TreatAsAtomicUnit=on
  Read_Gyro16 : Subsystem  TreatAsAtomicUnit=on
  Read_Gyro9 : Subsystem  TreatAsAtomicUnit=on
  wires:
  In1/1 -> Compare To Constant8/1, Compare To Constant10/1, Compare To Constant12/1, Compare To Constant13/1, Compare To Constant14/1, Compare To Constant15/1, Compare To Constant16/1, Compare To Constant17/1
  Compare To Constant8/1 -> Read_Gyro9/Trigger
  Compare To Constant12/1 -> Read_Gyro11/Trigger
  Compare To Constant17/1 -> Read_Gyro16/Trigger
  Compare To Constant16/1 -> Read_Gyro15/Trigger
  Compare To Constant14/1 -> Read_Gyro13/Trigger
  Compare To Constant10/1 -> Read_Gyro10/Trigger
  Compare To Constant13/1 -> Read_Gyro12/Trigger
  Compare To Constant15/1 -> Read_Gyro14/Trigger

== system Charge_2_V1/HANcoder STM32 Target - E407-STM32 algorithm/Energy Meter1/Energymeter_Request/Fequency ==
  In1 : Inport
  Compare To Constant10 : simulink/Logic and Bit Operations/Compare To Constant  relop===  const=402  OutDataTypeStr=boolean
  Compare To Constant12 : simulink/Logic and Bit Operations/Compare To Constant  relop===  const=403  OutDataTypeStr=boolean
  Compare To Constant13 : simulink/Logic and Bit Operations/Compare To Constant  relop===  const=404  OutDataTypeStr=boolean
  Compare To Constant14 : simulink/Logic and Bit Operations/Compare To Constant  relop===  const=405  OutDataTypeStr=boolean
  Compare To Constant15 : simulink/Logic and Bit Operations/Compare To Constant  relop===  const=406  OutDataTypeStr=boolean
  Compare To Constant16 : simulink/Logic and Bit Operations/Compare To Constant  relop===  const=407  OutDataTypeStr=boolean
  Compare To Constant17 : simulink/Logic and Bit Operations/Compare To Constant  relop===  const=408  OutDataTypeStr=boolean
  Compare To Constant8 : simulink/Logic and Bit Operations/Compare To Constant  relop===  const=401  OutDataTypeStr=boolean
  Read_Gyro10 : Subsystem  TreatAsAtomicUnit=on
  Read_Gyro11 : Subsystem  TreatAsAtomicUnit=on
  Read_Gyro12 : Subsystem  TreatAsAtomicUnit=on
  Read_Gyro13 : Subsystem  TreatAsAtomicUnit=on
  Read_Gyro14 : Subsystem  TreatAsAtomicUnit=on
  Read_Gyro15 : Subsystem  TreatAsAtomicUnit=on
  Read_Gyro16 : Subsystem  TreatAsAtomicUnit=on
  Read_Gyro9 : Subsystem  TreatAsAtomicUnit=on
  wires:
  Compare To Constant15/1 -> Read_Gyro14/Trigger
  Compare To Constant13/1 -> Read_Gyro12/Trigger
  Compare To Constant10/1 -> Read_Gyro10/Trigger
  Compare To Constant14/1 -> Read_Gyro13/Trigger
  Compare To Constant16/1 -> Read_Gyro15/Trigger
  Compare To Constant17/1 -> Read_Gyro16/Trigger
  Compare To Constant12/1 -> Read_Gyro11/Trigger
  Compare To Constant8/1 -> Read_Gyro9/Trigger
  In1/1 -> Compare To Constant8/1, Compare To Constant17/1, Compare To Constant16/1, Compare To Constant15/1, Compare To Constant14/1, Compare To Constant13/1, Compare To Constant12/1, Compare To Constant10/1

== system Charge_2_V1/HANcoder STM32 Target - E407-STM32 algorithm/Energy Meter1/Energymeter_Request/RequestMessages_Enable  ==
  In1 : Inport
  Constant : Constant  OutDataTypeStr=boolean  SampleTime=-1
  Constant1 : Constant  Value=0  OutDataTypeStr=boolean  SampleTime=-1
  Digital Output : HANcoder_STM32_Target/STM32-E407/Digital Outputs/Digital Output  Tag=HANcoder_TARGET_STM32_E407  pinID=CON PD - 7  config=Push pull  tsamp=-1
      settings: SourceProductName=HANcoder STM32 Target
  Logical Operator1 : Logic  Operator=OR  Inputs=5  AllPortsSameDT=off  OutDataTypeStr=boolean
  Subsystem : Subsystem
  Subsystem1 : Subsystem
  Subsystem2 : Subsystem
  Subsystem3 : Subsystem
  Subsystem4 : Subsystem
  Switch : Switch  Criteria=u2 > Threshold
  wires:
  Logical Operator1/1 -> Switch/2
  Constant1/1 -> Switch/3
  Constant/1 -> Switch/1
  Switch/1 -> Digital Output/1  "enable"
  In1/1 -> Subsystem4/1(In1), Subsystem3/1(In1), Subsystem2/1(In1), Subsystem1/1(In1), Subsystem/1(In1)
  Subsystem/1(Out1) -> Logical Operator1/1
  Subsystem1/1(Out1) -> Logical Operator1/2
  Subsystem2/1(Out1) -> Logical Operator1/3
  Subsystem4/1(Out1) -> Logical Operator1/5
  Subsystem3/1(Out1) -> Logical Operator1/4

== system Charge_2_V1/HANcoder STM32 Target - E407-STM32 algorithm/Energy Meter1/Energymeter_Request/Voltage_meter_1 ==
  In1 : Inport
  Compare To Constant : simulink/Logic and Bit Operations/Compare To Constant  relop===  const=601  OutDataTypeStr=boolean
  Compare To Constant1 : simulink/Logic and Bit Operations/Compare To Constant  relop===  const=602  OutDataTypeStr=boolean
  Compare To Constant2 : simulink/Logic and Bit Operations/Compare To Constant  relop===  const=603  OutDataTypeStr=boolean
  Compare To Constant3 : simulink/Logic and Bit Operations/Compare To Constant  relop===  const=604  OutDataTypeStr=boolean
  Compare To Constant4 : simulink/Logic and Bit Operations/Compare To Constant  relop===  const=605  OutDataTypeStr=boolean
  Compare To Constant5 : simulink/Logic and Bit Operations/Compare To Constant  relop===  const=606  OutDataTypeStr=boolean
  Compare To Constant6 : simulink/Logic and Bit Operations/Compare To Constant  relop===  const=607  OutDataTypeStr=boolean
  Compare To Constant7 : simulink/Logic and Bit Operations/Compare To Constant  relop===  const=608  OutDataTypeStr=boolean
  Read_Gyro1 : Subsystem  TreatAsAtomicUnit=on
  Read_Gyro2 : Subsystem  TreatAsAtomicUnit=on
  Read_Gyro3 : Subsystem  TreatAsAtomicUnit=on
  Read_Gyro4 : Subsystem  TreatAsAtomicUnit=on
  Read_Gyro5 : Subsystem  TreatAsAtomicUnit=on
  Read_Gyro6 : Subsystem  TreatAsAtomicUnit=on
  Read_Gyro7 : Subsystem  TreatAsAtomicUnit=on
  Read_Gyro8 : Subsystem  TreatAsAtomicUnit=on
  wires:
  Compare To Constant3/1 -> Read_Gyro4/Trigger
  Compare To Constant1/1 -> Read_Gyro2/Trigger
  Compare To Constant2/1 -> Read_Gyro3/Trigger
  Compare To Constant/1 -> Read_Gyro1/Trigger
  Compare To Constant4/1 -> Read_Gyro5/Trigger
  Compare To Constant5/1 -> Read_Gyro6/Trigger
  Compare To Constant6/1 -> Read_Gyro7/Trigger
  Compare To Constant7/1 -> Read_Gyro8/Trigger
  In1/1 -> Compare To Constant/1, Compare To Constant1/1, Compare To Constant2/1, Compare To Constant3/1, Compare To Constant4/1, Compare To Constant5/1, Compare To Constant6/1, Compare To Constant7/1

== system Charge_2_V1/HANcoder STM32 Target - E407-STM32 algorithm/Energy Meter1/Energymeter_Request/Voltage_meter_2 ==
  In1 : Inport
  Compare To Constant : simulink/Logic and Bit Operations/Compare To Constant  relop===  const=801  OutDataTypeStr=boolean
  Compare To Constant1 : simulink/Logic and Bit Operations/Compare To Constant  relop===  const=802  OutDataTypeStr=boolean
  Compare To Constant2 : simulink/Logic and Bit Operations/Compare To Constant  relop===  const=803  OutDataTypeStr=boolean
  Compare To Constant3 : simulink/Logic and Bit Operations/Compare To Constant  relop===  const=804  OutDataTypeStr=boolean
  Compare To Constant4 : simulink/Logic and Bit Operations/Compare To Constant  relop===  const=805  OutDataTypeStr=boolean
  Compare To Constant5 : simulink/Logic and Bit Operations/Compare To Constant  relop===  const=806  OutDataTypeStr=boolean
  Compare To Constant6 : simulink/Logic and Bit Operations/Compare To Constant  relop===  const=807  OutDataTypeStr=boolean
  Compare To Constant7 : simulink/Logic and Bit Operations/Compare To Constant  relop===  const=808  OutDataTypeStr=boolean
  Read_Gyro1 : Subsystem  TreatAsAtomicUnit=on
  Read_Gyro2 : Subsystem  TreatAsAtomicUnit=on
  Read_Gyro3 : Subsystem  TreatAsAtomicUnit=on
  Read_Gyro4 : Subsystem  TreatAsAtomicUnit=on
  Read_Gyro5 : Subsystem  TreatAsAtomicUnit=on
  Read_Gyro6 : Subsystem  TreatAsAtomicUnit=on
  Read_Gyro7 : Subsystem  TreatAsAtomicUnit=on
  Read_Gyro8 : Subsystem  TreatAsAtomicUnit=on
  wires:
  In1/1 -> Compare To Constant7/1, Compare To Constant6/1, Compare To Constant5/1, Compare To Constant4/1, Compare To Constant3/1, Compare To Constant2/1, Compare To Constant1/1, Compare To Constant/1
  Compare To Constant7/1 -> Read_Gyro8/Trigger
  Compare To Constant6/1 -> Read_Gyro7/Trigger
  Compare To Constant5/1 -> Read_Gyro6/Trigger
  Compare To Constant4/1 -> Read_Gyro5/Trigger
  Compare To Constant/1 -> Read_Gyro1/Trigger
  Compare To Constant2/1 -> Read_Gyro3/Trigger
  Compare To Constant1/1 -> Read_Gyro2/Trigger
  Compare To Constant3/1 -> Read_Gyro4/Trigger

== system Charge_2_V1/HANcoder STM32 Target - E407-STM32 algorithm/Energy Meter1/Particle/UART init ==
  Level-2 M-file S-Function : M-S-Function  FunctionName=sfcn_uart_init
  Term1 : Terminator
  wires:
  Level-2 M-file S-Function/1 -> Term1/1

== system Charge_2_V1/HANcoder STM32 Target - E407-STM32 algorithm/Partclie_SP_Receive/SP1/Read_Gyro ==
  Trigger : TriggerPort  VariantControl=Variant
  UART receive : Subsystem  AncestorBlock=HANcoder_STM32_Target/STM32-E407/UART/UART receive  mask(UART receive){channel=UART1: Con. 3-D1 & Con. 3-D0 (PB6 & PB7), useStatusOut=off, tsamp=-1}
      mask prompts: useStatusOut "Use status outport"; tsamp "Sample time"
      mask help:
      | Function
      | ==========
      | Reads a byte from the UART reception buffer.
      |
      | Parameters per channel
      | ======================
      | - Select channel
      | - Select if the status output should be enabled.
      |
      | Outputs
      | =======
      | - The value of the receive byte.
      | - When the status output is 0, the reception buffer was empty.
      mask init:
      | uartChannelInfoStr = sfcn_uart_receive_mcb(2, channel, useStatusOut);
      settings: MoveFcn=drawLogos
      mask Help: web('sfcn_uart_receive.html')
      mask TypeOptions channel: UART1: Con. 3-D1 & Con. 3-D0 (PB6 & PB7) | UART2: Con. PD-8 & Con. PD-9 (PD5 & PD6) | UART3: Con. PD-11 & Con. PD-12 (PD8 & PD9) | UART6: Con. UEXT-3 & Con. UEXT-4 (PC6 & PC7)
      mask Display: fprintf('UART receive\n%s', uartChannelInfoStr);patch([240 246 246],[8 14 2],[1 0 0]);patch([248 248 254],[14 2 8],[0 0 0.35]);
  Out1 : Outport
  wires:
  UART receive/1(Out1) -> Out1/1

== system Charge_2_V1/HANcoder STM32 Target - E407-STM32 algorithm/Partclie_SP_Receive/SP1/Read_Gyro1 ==
  Trigger : TriggerPort  VariantControl=Variant
  UART receive : Subsystem  AncestorBlock=HANcoder_STM32_Target/STM32-E407/UART/UART receive  mask(UART receive){channel=UART1: Con. 3-D1 & Con. 3-D0 (PB6 & PB7), useStatusOut=off, tsamp=-1}
      mask prompts: useStatusOut "Use status outport"; tsamp "Sample time"
      mask help:
      | Function
      | ==========
      | Reads a byte from the UART reception buffer.
      |
      | Parameters per channel
      | ======================
      | - Select channel
      | - Select if the status output should be enabled.
      |
      | Outputs
      | =======
      | - The value of the receive byte.
      | - When the status output is 0, the reception buffer was empty.
      mask init:
      | uartChannelInfoStr = sfcn_uart_receive_mcb(2, channel, useStatusOut);
      settings: MoveFcn=drawLogos
      mask Help: web('sfcn_uart_receive.html')
      mask TypeOptions channel: UART1: Con. 3-D1 & Con. 3-D0 (PB6 & PB7) | UART2: Con. PD-8 & Con. PD-9 (PD5 & PD6) | UART3: Con. PD-11 & Con. PD-12 (PD8 & PD9) | UART6: Con. UEXT-3 & Con. UEXT-4 (PC6 & PC7)
      mask Display: fprintf('UART receive\n%s', uartChannelInfoStr);patch([240 246 246],[8 14 2],[1 0 0]);patch([248 248 254],[14 2 8],[0 0 0.35]);
  Out1 : Outport
  wires:
  UART receive/1(Out1) -> Out1/1

== system Charge_2_V1/HANcoder STM32 Target - E407-STM32 algorithm/Partclie_SP_Receive/SP1/Read_Gyro2 ==
  Trigger : TriggerPort  VariantControl=Variant
  UART receive : Subsystem  AncestorBlock=HANcoder_STM32_Target/STM32-E407/UART/UART receive  mask(UART receive){channel=UART1: Con. 3-D1 & Con. 3-D0 (PB6 & PB7), useStatusOut=off, tsamp=-1}
      mask prompts: useStatusOut "Use status outport"; tsamp "Sample time"
      mask help:
      | Function
      | ==========
      | Reads a byte from the UART reception buffer.
      |
      | Parameters per channel
      | ======================
      | - Select channel
      | - Select if the status output should be enabled.
      |
      | Outputs
      | =======
      | - The value of the receive byte.
      | - When the status output is 0, the reception buffer was empty.
      mask init:
      | uartChannelInfoStr = sfcn_uart_receive_mcb(2, channel, useStatusOut);
      settings: MoveFcn=drawLogos
      mask Help: web('sfcn_uart_receive.html')
      mask TypeOptions channel: UART1: Con. 3-D1 & Con. 3-D0 (PB6 & PB7) | UART2: Con. PD-8 & Con. PD-9 (PD5 & PD6) | UART3: Con. PD-11 & Con. PD-12 (PD8 & PD9) | UART6: Con. UEXT-3 & Con. UEXT-4 (PC6 & PC7)
      mask Display: fprintf('UART receive\n%s', uartChannelInfoStr);patch([240 246 246],[8 14 2],[1 0 0]);patch([248 248 254],[14 2 8],[0 0 0.35]);
  Out1 : Outport
  wires:
  UART receive/1(Out1) -> Out1/1

== system Charge_2_V1/HANcoder STM32 Target - E407-STM32 algorithm/Partclie_SP_Receive/SP1/Read_Gyro3 ==
  Trigger : TriggerPort  VariantControl=Variant
  UART receive : Subsystem  AncestorBlock=HANcoder_STM32_Target/STM32-E407/UART/UART receive  mask(UART receive){channel=UART1: Con. 3-D1 & Con. 3-D0 (PB6 & PB7), useStatusOut=off, tsamp=-1}
      mask prompts: useStatusOut "Use status outport"; tsamp "Sample time"
      mask help:
      | Function
      | ==========
      | Reads a byte from the UART reception buffer.
      |
      | Parameters per channel
      | ======================
      | - Select channel
      | - Select if the status output should be enabled.
      |
      | Outputs
      | =======
      | - The value of the receive byte.
      | - When the status output is 0, the reception buffer was empty.
      mask init:
      | uartChannelInfoStr = sfcn_uart_receive_mcb(2, channel, useStatusOut);
      settings: MoveFcn=drawLogos
      mask Help: web('sfcn_uart_receive.html')
      mask TypeOptions channel: UART1: Con. 3-D1 & Con. 3-D0 (PB6 & PB7) | UART2: Con. PD-8 & Con. PD-9 (PD5 & PD6) | UART3: Con. PD-11 & Con. PD-12 (PD8 & PD9) | UART6: Con. UEXT-3 & Con. UEXT-4 (PC6 & PC7)
      mask Display: fprintf('UART receive\n%s', uartChannelInfoStr);patch([240 246 246],[8 14 2],[1 0 0]);patch([248 248 254],[14 2 8],[0 0 0.35]);
  Out1 : Outport
  wires:
  UART receive/1(Out1) -> Out1/1

== system Charge_2_V1/HANcoder STM32 Target - E407-STM32 algorithm/Partclie_SP_Receive/SP1/Subsystem ==
  In1 : Inport
  In2 : Inport  Port=2
  In3 : Inport  Port=3
  Setpoint1 : Inport  Port=4
  In5 : Inport  Port=5
  In6 : Inport  Port=6
  Delay : Delay  DelayLength=1  InitialCondition=0
  Delay1 : Delay  DelayLength=1  InitialCondition=0
  Delay2 : Delay  DelayLength=1  InitialCondition=0
  Logical Operator : Logic  Inputs=4  AllPortsSameDT=off  OutDataTypeStr=boolean
  Logical Operator1 : Logic  Operator=OR  AllPortsSameDT=off  OutDataTypeStr=boolean
  Switch : Switch  Criteria=u2 > Threshold
  Switch1 : Switch  Criteria=u2 > Threshold
  Switch2 : Switch  Criteria=u2 > Threshold
  SP1_P : Outport
  SP2_P : Outport  Port=2
  wires:
  Logical Operator1/1 -> Logical Operator/2
  In6/1 -> Logical Operator/4
  Switch2/1 -> SP2_P/1, Delay2/1  "SP2_P"
  In3/1 -> Switch2/2, Logical Operator1/2
  Logical Operator/1 -> Switch/2
  Switch/1 -> Switch1/1, Delay/1, Switch2/1
  Delay/1 -> Switch/3
  In5/1 -> Logical Operator/3
  In2/1 -> Switch1/2, Logical Operator1/1
  In1/1 -> Logical Operator/1
  Setpoint1/1 -> Switch/1
  Delay1/1 -> Switch1/3
  Delay2/1 -> Switch2/3
  Switch1/1 -> SP1_P/1, Delay1/1  "SP1_P"

== system Charge_2_V1/HANcoder STM32 Target - E407-STM32 algorithm/Car1/Pilotcar1/Max_filter/If Action Subsystem ==
  In1 : Inport
  Action Port : ActionPort  ActionType=then
  Out1 : Outport
  wires:
  In1/1 -> Out1/1

== system Charge_2_V1/HANcoder STM32 Target - E407-STM32 algorithm/Car1/Pilotcar1/Max_filter/If Action Subsystem1 ==
  In1 : Inport
  Action Port : ActionPort  ActionType=else
  Out1 : Outport
  wires:
  In1/1 -> Out1/1

== system Charge_2_V1/HANcoder STM32 Target - E407-STM32 algorithm/Car1/Pilotcar1/Min_filter/If Action Subsystem2 ==
  In1 : Inport
  Action Port : ActionPort  ActionType=then
  Out1 : Outport
  wires:
  In1/1 -> Out1/1

== system Charge_2_V1/HANcoder STM32 Target - E407-STM32 algorithm/Car1/Pilotcar1/Min_filter/If Action Subsystem3 ==
  In1 : Inport
  Action Port : ActionPort  ActionType=else
  Out1 : Outport
  wires:
  In1/1 -> Out1/1

== system Charge_2_V1/HANcoder STM32 Target - E407-STM32 algorithm/Car2/Pilotcar2/Max_filter/If Action Subsystem ==
  In1 : Inport
  Action Port : ActionPort  ActionType=then
  Out1 : Outport
  wires:
  In1/1 -> Out1/1

== system Charge_2_V1/HANcoder STM32 Target - E407-STM32 algorithm/Car2/Pilotcar2/Max_filter/If Action Subsystem1 ==
  In1 : Inport
  Action Port : ActionPort  ActionType=else
  Out1 : Outport
  wires:
  In1/1 -> Out1/1

== system Charge_2_V1/HANcoder STM32 Target - E407-STM32 algorithm/Car2/Pilotcar2/Min_filter/If Action Subsystem2 ==
  In1 : Inport
  Action Port : ActionPort  ActionType=then
  Out1 : Outport
  wires:
  In1/1 -> Out1/1

== system Charge_2_V1/HANcoder STM32 Target - E407-STM32 algorithm/Car2/Pilotcar2/Min_filter/If Action Subsystem3 ==
  In1 : Inport
  Action Port : ActionPort  ActionType=else
  Out1 : Outport
  wires:
  In1/1 -> Out1/1

== system Charge_2_V1/HANcoder STM32 Target - E407-STM32 algorithm/Current_SP/Subsystem1/Fre_Control/16A_Car ==
  Fre : Inport
  Add : Sum
  Add{1..2,4..5} (4 alike) : Sum  Inputs=+-
  Add3 : Sum
  Constant : Constant  Value=10  OutDataTypeStr=single  SampleTime=-1
  Constant1 : Constant  Value=6  OutDataTypeStr=single  SampleTime=-1
  Constant2 : Constant  Value=6  OutDataTypeStr=single  SampleTime=-1
  Constant3 : Constant  Value=Frequency_Low_Point  OutDataTypeStr=single  SampleTime=-1
  Constant4 : Constant  Value=16  OutDataTypeStr=single  SampleTime=-1
  Constant5 : Constant  Value=Frequency_Mid_high  OutDataTypeStr=single  SampleTime=-1
  Product : Product
  Product1 : Product
  Out1 : Outport
  Out2 : Outport  Port=2
  Out3 : Outport  Port=3
  wires:
  Fre/1 -> Add2/1, Add5/1
  Constant4/1 -> Add4/1
  Add3/1 -> Out3/1
  Add/1 -> Out1/1
  Add5/1 -> Product1/2
  Product1/1 -> Add3/1
  Add2/1 -> Product/2
  Constant3/1 -> Add2/2
  Constant5/1 -> Add5/2
  Product/1 -> Add/1
  Constant/1 -> Add1/1, Out2/1, Add4/2, Add3/2
  Constant2/1 -> Add1/2
  Add1/1 -> Product/1
  Add4/1 -> Product1/1
  Constant1/1 -> Add/2

== system Charge_2_V1/HANcoder STM32 Target - E407-STM32 algorithm/Current_SP/Subsystem1/Fre_Control/32A_Car1 ==
  fre : Inport
  Add : Sum
  Add{1..2,4..5} (4 alike) : Sum  Inputs=+-
  Add3 : Sum
  Constant : Constant  Value=24  OutDataTypeStr=single  SampleTime=-1
  Constant1 : Constant  Value=6  OutDataTypeStr=single  SampleTime=-1
  Constant2 : Constant  Value=6  OutDataTypeStr=single  SampleTime=-1
  Constant3 : Constant  Value=Frequency_Low_Point  OutDataTypeStr=single  SampleTime=-1
  Constant4 : Constant  Value=32  OutDataTypeStr=single  SampleTime=-1
  Constant5 : Constant  Value=Frequency_Mid_high  OutDataTypeStr=single  SampleTime=-1
  Product : Product
  Product1 : Product
  Out1 : Outport
  Out2 : Outport  Port=2
  Out3 : Outport  Port=3
  wires:
  Constant1/1 -> Add/2
  Add4/1 -> Product1/1
  Add1/1 -> Product/1
  Constant2/1 -> Add1/2
  Constant/1 -> Add4/2, Add3/2, Add1/1, Out2/1
  Product/1 -> Add/1
  Constant5/1 -> Add5/2
  Constant3/1 -> Add2/2
  Add2/1 -> Product/2
  Product1/1 -> Add3/1
  Add5/1 -> Product1/2
  Add/1 -> Out1/1
  Add3/1 -> Out3/1
  Constant4/1 -> Add4/1
  fre/1 -> Add5/1, Add2/1
